simulink model "FlightSimulator_4160MODS"  (R2018a)
settings: Solver=FixedStepAuto  StartTime=0.0  StopTime=inf  RelTol=1e-3  EnableMultiTasking=on
undefined symbols (not defined in the file): LF, serial
libraries: aerolibutil x5, simulink x3, instrumentlib x3, sharedtransform x2, hdlsllib x1
settings Model: SimulationMode=accelerator  EnablePacing=on  PacingRate=1000  ExtModeTrigDuration=2  ExplicitPartitioning=on  Creator=argue  LastModifiedBy=User
settings OptimizationCC: EnhancedBackFolding=on  PassReuseOutputArgsAs=Individual arguments  MaxStackSize=64  OptimizeBlockOrder=speed  DifferentSizesBufferReuse=on  OptimizationCustomize=off
settings DebuggingCC: ParameterTunabilityLossMsg=error
settings HardwareCC: ProdBitPerPointer=32  ProdBitPerSizeT=32  ProdBitPerPtrDiffT=32  ProdLargestAtomicInteger=Long  ProdLargestAtomicFloat=Double  ProdWordSize=32  ProdHWDeviceType=ARM Compatible->ARM Cortex
settings SFSimCC: MATLABDynamicMemAlloc=off
settings RTWCC: SystemTargetFile=ert.tlc  HardwareBoard=Arduino Due  TLCOptions=-aInlineSetEventsForThisBaseRateFcn=TLC_FALSE -aSuppressMultiTaskScheduler=TLC_FALSE -aRateBasedStepFcn=1  TemplateMakefile=ert_default_tmf  GenerateReport=on  Toolchain=Arduino ARM  BuildConfiguration=Faster Runs  IncludeHyperlinkInReport=on  LaunchReport=on  GenerateTraceInfo=on  GenerateTraceReport=on  GenerateTraceReportSl=on  GenerateTraceReportSf=on  GenerateTraceReportEml=on
settings CodeAppCC: ForceParamTrailComments=on  IgnoreCustomStorageClasses=off  OperatorAnnotations=on  SimulinkDataObjDesc=on  SFDataObjDesc=on  InsertBlockDesc=on
settings ERTTargetCC: SupportContinuousTime=on  SupportVariableSizeSignals=on

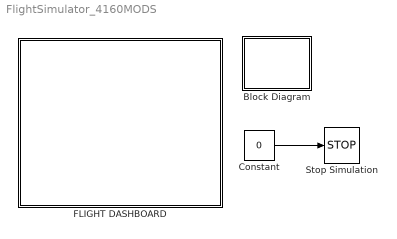
== system FlightSimulator_4160MODS ==
  Block Diagram : Subsystem
  Constant : Constant  Value=0
  FLIGHT DASHBOARD : Subsystem
  Stop Simulation : Stop
  wires:
  Constant/1 -> Stop Simulation/1

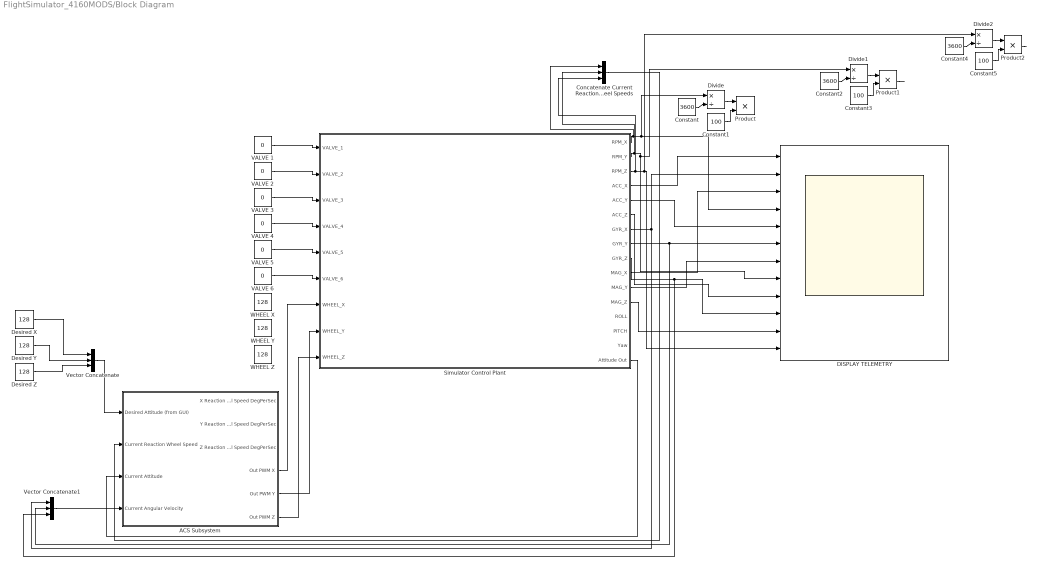
== system FlightSimulator_4160MODS/Block Diagram ==
  ACS Subsystem : Subsystem
  Concatenate Current Reaction Wheel Speeds : Concatenate  NumInputs=3
  Constant : Constant  Value=3600
  Constant1 : Constant  Value=100
  Constant2 : Constant  Value=3600
  Constant3 : Constant  Value=100
  Constant4 : Constant  Value=3600
  Constant5 : Constant  Value=100
  DISPLAY TELEMETRY : Scope  NumInputPorts=12
  Desired X : Constant  Value=128  OutDataTypeStr=double  SampleTime=-1
  Desired Y : Constant  Value=128  OutDataTypeStr=double  SampleTime=-1
  Desired Z : Constant  Value=128  OutDataTypeStr=double  SampleTime=-1
  Divide : Product  Inputs=*/
  Divide1 : Product  Inputs=*/
  Divide2 : Product  Inputs=*/
  Product : Product
  Product1 : Product
  Product2 : Product
  Simulator Control Plant : Subsystem
  VALVE {1..6} (6 alike) : Constant  Value=0  SampleTime=0.01
  Vector Concatenate : Concatenate  NumInputs=3
  Vector Concatenate1 : Concatenate  NumInputs=3
  WHEEL X : Constant  Value=128  OutDataTypeStr=int16  SampleTime=-1
  WHEEL Y : Constant  Value=128  OutDataTypeStr=int16  SampleTime=-1
  WHEEL Z : Constant  Value=128  OutDataTypeStr=int16  SampleTime=-1
  wires:
  VALVE 6/1 -> Simulator Control Plant/6(VALVE_6)
  VALVE 2/1 -> Simulator Control Plant/2(VALVE_2)
  VALVE 3/1 -> Simulator Control Plant/3(VALVE_3)
  VALVE 5/1 -> Simulator Control Plant/5(VALVE_5)
  VALVE 1/1 -> Simulator Control Plant/1(VALVE_1)
  VALVE 4/1 -> Simulator Control Plant/4(VALVE_4)
  Simulator Control Plant/4(" ACC_X") -> DISPLAY TELEMETRY/1
  Simulator Control Plant/7(GYR_X) -> Vector Concatenate1/1, DISPLAY TELEMETRY/2
  Simulator Control Plant/10(MAG_X) -> DISPLAY TELEMETRY/3
  Simulator Control Plant/1(RPM_X) -> Concatenate Current Reaction Wheel Speeds/1, Divide/1, DISPLAY TELEMETRY/4
  Simulator Control Plant/5(" ACC_Y") -> DISPLAY TELEMETRY/5
  Simulator Control Plant/8(GYR_Y) -> Vector Concatenate1/2, DISPLAY TELEMETRY/6
  Simulator Control Plant/11(MAG_Y) -> DISPLAY TELEMETRY/7
  Simulator Control Plant/6(" ACC_Z") -> DISPLAY TELEMETRY/9
  Simulator Control Plant/9(GYR_Z) -> Vector Concatenate1/3, DISPLAY TELEMETRY/10
  Simulator Control Plant/12(MAG_Z) -> DISPLAY TELEMETRY/11
  Constant/1 -> Divide/2
  Divide/1 -> Product/1
  Constant1/1 -> Product/2
  Simulator Control Plant/2(RPM_Y) -> Concatenate Current Reaction Wheel Speeds/2, Divide1/1, DISPLAY TELEMETRY/8
  Constant2/1 -> Divide1/2
  Divide1/1 -> Product1/1
  Constant3/1 -> Product1/2
  Divide2/1 -> Product2/1
  Constant4/1 -> Divide2/2
  Simulator Control Plant/3(RPM_Z) -> Concatenate Current Reaction Wheel Speeds/3, Divide2/1, DISPLAY TELEMETRY/12
  Constant5/1 -> Product2/2
  Product2/1 -> ?
  Product1/1 -> ?
  ACS Subsystem/6(Out PWM Z) -> Simulator Control Plant/9(WHEEL_Z)
  ACS Subsystem/5(Out PWM Y) -> Simulator Control Plant/8(WHEEL_Y)
  ACS Subsystem/4(Out PWM X) -> Simulator Control Plant/7(WHEEL_X)
  Concatenate Current Reaction Wheel Speeds/1 -> ACS Subsystem/2(Current Reaction Wheel Speed)
  Simulator Control Plant/16(" Attitude Out") -> ACS Subsystem/3(Current Attitude)
  Desired X/1 -> Vector Concatenate/1
  Desired Y/1 -> Vector Concatenate/2
  Desired Z/1 -> Vector Concatenate/3
  Vector Concatenate/1 -> ACS Subsystem/1(Desired Attitude (from GUI))
  Vector Concatenate1/1 -> ACS Subsystem/4(Current Angular Velocity)

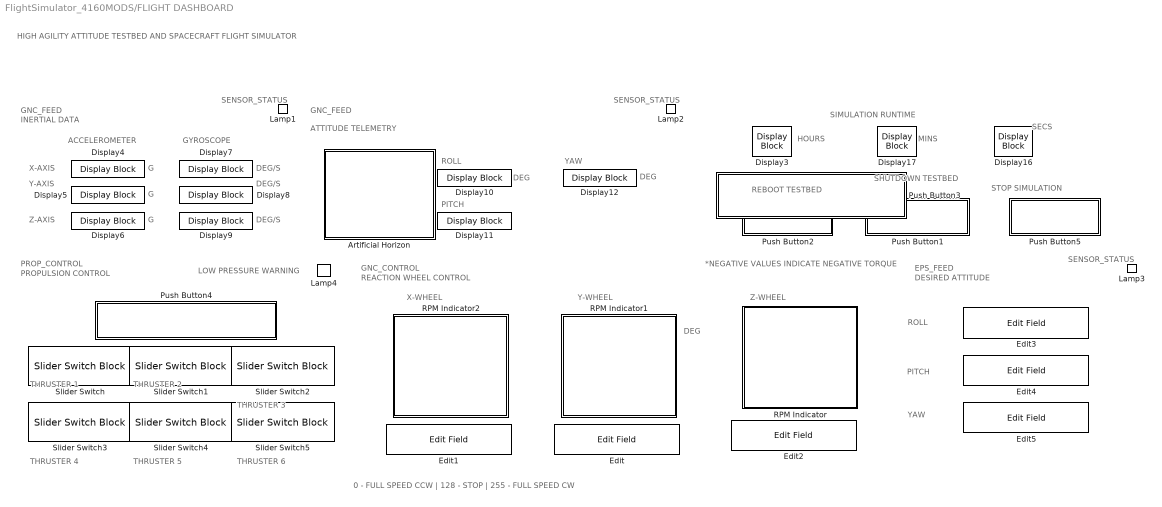
== system FlightSimulator_4160MODS/FLIGHT DASHBOARD ==
  note: HIGH AGILITY ATTITUDE TESTBED AND SPACECRAFT FLIGHT SIMULATOR
  note: PROPULSION CONTROL
  note: X-WHEEL
  note: LOW PRESSURE WARNING
  note: DESIRED ATTITUDE
  note: REACTION WHEEL CONTROL
  note: EPS_FEED
  note: PROP_CONTROL
  note: GNC_CONTROL
  note: GNC_FEED
  note: INERTIAL DATA
  note: G
  note: G
  note: G
  note: ACCELEROMETER
  note: X-AXIS
  note: Y-AXIS
  note: Z-AXIS
  note: GYROSCOPE
  note: DEG/S
  note: DEG/S
  note: DEG/S
  note: GNC_FEED
  note: ATTITUDE TELEMETRY
  note: ROLL
  note: PITCH
  note: YAW
  note: DEG
  note: DEG
  note: DEG
  note: SENSOR_STATUS
  note: SENSOR_STATUS
  note: SENSOR_STATUS
  note: *NEGATIVE VALUES INDICATE NEGATIVE TORQUE
  note: REBOOT TESTBED
  note: HOURS
  note: SECS
  note: MINS
  note: SIMULATION RUNTIME
  note: SHUTDOWN TESTBED
  note: STOP SIMULATION
  note: Y-WHEEL
  note: Z-WHEEL
  note: 0 - FULL SPEED CCW | 128 - STOP | 255 - FULL SPEED CW
  note: THRUSTER 1
  note: THRUSTER 2
  note: THRUSTER 3
  note: THRUSTER 4
  note: THRUSTER 6
  note: THRUSTER 5
  note: ROLL
  note: PITCH
  note: YAW
  Artificial Horizon : Subsystem  DialogController=aeroblksHMICreateDDGDialog  IsWebBlock=on  mask(MWDashboardBlock){webBlockId=87d256c6-158d-4fe2-b150-9c42d0428838, webBlockType=artificialhorizon, ShowInLibBrowser=on, ShowInitialText=on, HMISrcModelName=FlightSimulator}
      mask prompts: webBlockId "WebBlock Id"; webBlockType "WebBlock Type"; HMISrcModelName "Source Model"
      mask help: aeroblksHMI:aeroblkhmi:ArtificialHorizonDialogDesc
      mask Help: eval('asbhmihelp(''artificialhorizon'')');
      mask Display:
      | if strcmp(get_param(bdroot(gcb),'BlockDiagramType'), 'library')
      |  image([(matlabroot) '/toolbox/aeroblks/aeroblks/hmi/icons/ArtificialHorizonIcon.svg'])
      | end
  Display10 : DisplayBlock  WebBlockId=325  LabelPosition=Hide  Alignment=Left
  Display11 : DisplayBlock  WebBlockId=327  LabelPosition=Hide  Alignment=Left
  Display12 : DisplayBlock  WebBlockId=329  LabelPosition=Hide  Alignment=Left
  Display16 : DisplayBlock  WebBlockId=711  LabelPosition=Hide  Alignment=Left
  Display17 : DisplayBlock  WebBlockId=712  LabelPosition=Hide  Alignment=Left
  Display3 : DisplayBlock  WebBlockId=710  LabelPosition=Hide  Alignment=Left
  Display4 : DisplayBlock  WebBlockId=266  LabelPosition=Hide  Alignment=Left
  Display5 : DisplayBlock  WebBlockId=268  LabelPosition=Hide  Alignment=Left
  Display6 : DisplayBlock  WebBlockId=270  LabelPosition=Hide  Alignment=Left
  Display7 : DisplayBlock  WebBlockId=313  LabelPosition=Hide  Alignment=Left
  Display8 : DisplayBlock  WebBlockId=314  LabelPosition=Hide  Alignment=Left
  Display9 : DisplayBlock  WebBlockId=315  LabelPosition=Hide  Alignment=Left
  Edit : EditField  WebBlockId=830  LabelPosition=Hide  Alignment=Center
  Edit1 : EditField  WebBlockId=828  LabelPosition=Hide  Alignment=Center
  Edit2 : EditField  WebBlockId=829  LabelPosition=Hide  Alignment=Center
  Edit3 : EditField  WebBlockId=1336  LabelPosition=Hide  Alignment=Center
  Edit4 : EditField  WebBlockId=1337  LabelPosition=Hide  Alignment=Center
  Edit5 : EditField  WebBlockId=1338  LabelPosition=Hide  Alignment=Center
  Lamp1 : LampBlock  WebBlockId=841  LabelPosition=Hide
  Lamp2 : LampBlock  WebBlockId=399  LabelPosition=Hide
  Lamp3 : LampBlock  WebBlockId=401  LabelPosition=Hide
  Lamp4 : LampBlock  WebBlockId=1063  LabelPosition=Hide
  Push Button1 : Subsystem  DialogController=hmiCreateDDGDialog  IsWebBlock=on  mask(MWDashboardBlock){webBlockId=5529e01b-399f-4366-a248-23a197ffef9f, webBlockType=pushbutton, ShowInLibBrwoser=on, ShowInitialText=on, HMISrcModelName=FlightSimulator}
      mask prompts: webBlockId "WebBlock Id"; webBlockType "WebBlock Type"; HMISrcModelName "Source Model"
      mask help: SimulinkHMI:dialogs:PushButtonDialogDesc
      mask Help: helpview([docroot '/mapfiles/simulink.map'], 'hmi_push_button')
      mask Display:
      | model = bdroot(gcb);
      | if strcmp(get_param(model,'BlockDiagramType'), 'library')
      |     image([(matlabroot) '/toolbox/simulink/hmi/icons/PushButton.png']);
      | end
  Push Button2 : Subsystem  DialogController=hmiCreateDDGDialog  IsWebBlock=on  mask(MWDashboardBlock){webBlockId=2e9611f3-365a-4a15-a648-271fb47c7cf3, webBlockType=pushbutton, ShowInLibBrwoser=on, ShowInitialText=on, HMISrcModelName=FlightSimulator}
      mask prompts: webBlockId "WebBlock Id"; webBlockType "WebBlock Type"; HMISrcModelName "Source Model"
      mask help: SimulinkHMI:dialogs:PushButtonDialogDesc
      mask Help: helpview([docroot '/mapfiles/simulink.map'], 'hmi_push_button')
      mask Display:
      | model = bdroot(gcb);
      | if strcmp(get_param(model,'BlockDiagramType'), 'library')
      |     image([(matlabroot) '/toolbox/simulink/hmi/icons/PushButton.png']);
      | end
  Push Button3 : Subsystem  DialogController=hmiCreateDDGDialog  IsWebBlock=on  mask(MWDashboardBlock){webBlockId=2b20586d-f367-4741-bf9b-3cb173f58035, webBlockType=pushbutton, ShowInLibBrowser=on, ShowInitialText=on, HMISrcModelName=FlightSimulator}
      mask prompts: webBlockId "WebBlock Id"; webBlockType "WebBlock Type"; HMISrcModelName "Source Model"
      mask help: Set a value of a tunable parameter or variable by selecting and holding the button. When the push button is not selected, the value is set back to the default value.
      mask Help: helpview([docroot '/mapfiles/simulink.map'], 'hmi_pushbutton')
      mask Display:
      | if strcmp(get_param(bdroot(gcb),'BlockDiagramType'),'library')
      |  image([(matlabroot) '/toolbox/simulink/hmi/icons/PushButton.png'])
      | end
  Push Button4 : Subsystem  DialogController=hmiCreateDDGDialog  IsWebBlock=on  mask(MWDashboardBlock){webBlockId=373ea6f1-33bb-479d-964f-0db2d45018c2, webBlockType=pushbutton, ShowInLibBrwoser=on, ShowInitialText=on, HMISrcModelName=FlightSimulator}
      mask prompts: webBlockId "WebBlock Id"; webBlockType "WebBlock Type"; HMISrcModelName "Source Model"
      mask help: SimulinkHMI:dialogs:PushButtonDialogDesc
      mask Help: helpview([docroot '/mapfiles/simulink.map'], 'hmi_push_button')
      mask Display:
      | model = bdroot(gcb);
      | if strcmp(get_param(model,'BlockDiagramType'), 'library')
      |     image([(matlabroot) '/toolbox/simulink/hmi/icons/PushButton.png']);
      | end
  Push Button5 : Subsystem  DialogController=hmiCreateDDGDialog  IsWebBlock=on  mask(MWDashboardBlock){webBlockId=d7fbd1aa-2ff5-4984-a2a7-416a94e4d3e9, webBlockType=pushbutton, ShowInLibBrwoser=on, ShowInitialText=on, HMISrcModelName=FlightSimulator}
      mask prompts: webBlockId "WebBlock Id"; webBlockType "WebBlock Type"; HMISrcModelName "Source Model"
      mask help: SimulinkHMI:dialogs:PushButtonDialogDesc
      mask Help: helpview([docroot '/mapfiles/simulink.map'], 'hmi_push_button')
      mask Display:
      | model = bdroot(gcb);
      | if strcmp(get_param(model,'BlockDiagramType'), 'library')
      |     image([(matlabroot) '/toolbox/simulink/hmi/icons/PushButton.png']);
      | end
  RPM Indicator : Subsystem  DialogController=aeroblksHMICreateDDGDialog  IsWebBlock=on  mask(MWDashboardBlock){webBlockId=08a9e829-d632-43db-b174-ac85f5d525a0, webBlockType=rpmindicator, ShowInLibBrowser=on, ShowInitialText=on, HMISrcModelName=FlightSimulator}
      mask prompts: webBlockId "WebBlock Id"; webBlockType "WebBlock Type"; HMISrcModelName "Source Model"
      mask help: aeroblksHMI:aeroblkhmi:RPMIndicatorDialogDesc
      mask Help: eval('asbhmihelp(''rpmindicator'')')
      mask Display:
      | if strcmp(get_param(bdroot(gcb),'BlockDiagramType'), 'library')
      |  image([(matlabroot) '/toolbox/aeroblks/aeroblks/hmi/icons/RPMIndicatorIcon.svg'])
      | end
  RPM Indicator1 : Subsystem  DialogController=aeroblksHMICreateDDGDialog  IsWebBlock=on  mask(MWDashboardBlock){webBlockId=8ce8b2ac-7bb7-4973-85b6-cdafd251f30d, webBlockType=rpmindicator, ShowInLibBrowser=on, ShowInitialText=on, HMISrcModelName=FlightSimulator}
      mask prompts: webBlockId "WebBlock Id"; webBlockType "WebBlock Type"; HMISrcModelName "Source Model"
      mask help: aeroblksHMI:aeroblkhmi:RPMIndicatorDialogDesc
      mask Help: eval('asbhmihelp(''rpmindicator'')')
      mask Display:
      | if strcmp(get_param(bdroot(gcb),'BlockDiagramType'), 'library')
      |  image([(matlabroot) '/toolbox/aeroblks/aeroblks/hmi/icons/RPMIndicatorIcon.svg'])
      | end
  RPM Indicator2 : Subsystem  DialogController=aeroblksHMICreateDDGDialog  IsWebBlock=on  mask(MWDashboardBlock){webBlockId=a80f6973-3156-4565-aff3-9397dcdba22e, webBlockType=rpmindicator, ShowInLibBrowser=on, ShowInitialText=on, HMISrcModelName=FlightSimulator}
      mask prompts: webBlockId "WebBlock Id"; webBlockType "WebBlock Type"; HMISrcModelName "Source Model"
      mask help: aeroblksHMI:aeroblkhmi:RPMIndicatorDialogDesc
      mask Help: eval('asbhmihelp(''rpmindicator'')')
      mask Display:
      | if strcmp(get_param(bdroot(gcb),'BlockDiagramType'), 'library')
      |  image([(matlabroot) '/toolbox/aeroblks/aeroblks/hmi/icons/RPMIndicatorIcon.svg'])
      | end
  Slider Switch : SliderSwitchBlock  WebBlockId=1066
      settings: Values={{'Off', 'On'}, [0 1]}
  Slider Switch1 : SliderSwitchBlock  WebBlockId=1067
      settings: Values={{'Off', 'On'}, [0 1]}
  Slider Switch2 : SliderSwitchBlock  WebBlockId=1068
      settings: Values={{'Off', 'On'}, [0 1]}
  Slider Switch3 : SliderSwitchBlock  WebBlockId=1069
      settings: Values={{'Off', 'On'}, [0 1]}
  Slider Switch4 : SliderSwitchBlock  WebBlockId=1070
      settings: Values={{'Off', 'On'}, [0 1]}
  Slider Switch5 : SliderSwitchBlock  WebBlockId=1071
      settings: Values={{'Off', 'On'}, [0 1]}

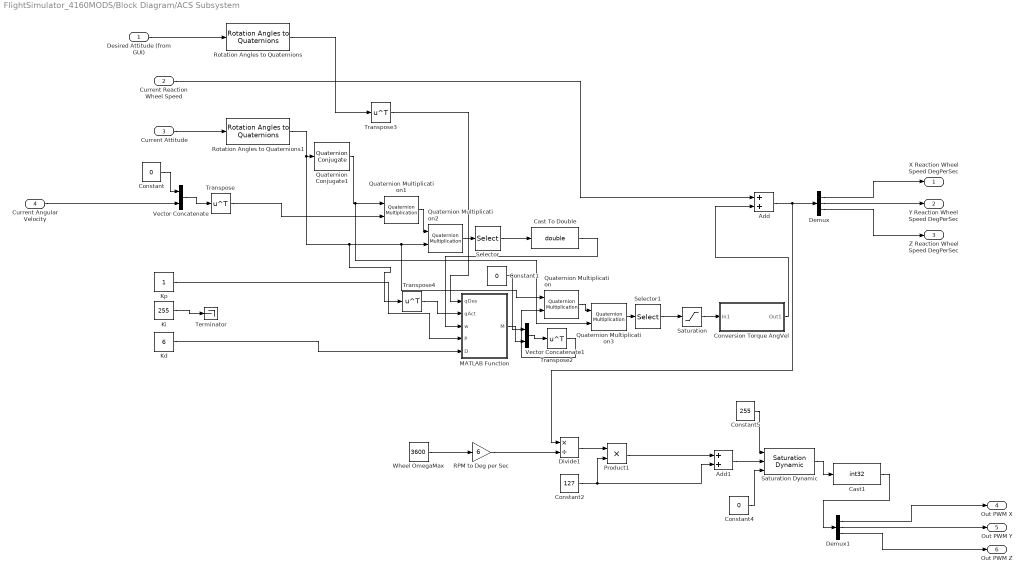
== system FlightSimulator_4160MODS/Block Diagram/ACS Subsystem ==
  Desired Attitude (from GUI) : Inport
  Current Reaction Wheel Speed : Inport  Port=2
  Current Attitude : Inport  Port=3
  Current Angular Velocity : Inport  Port=4
  Add : Sum
  Add1 : Sum
  Cast To Double : DataTypeConversion  OutDataTypeStr=double
  Cast1 : DataTypeConversion  OutDataTypeStr=int32  SaturateOnIntegerOverflow=on
  Constant : Constant  Value=0
  Constant1 : Constant  Value=0
  Constant2 : Constant  Value=127
  Constant4 : Constant  Value=0
  Constant5 : Constant  Value=255
  Conversion Torque AngVel : Subsystem
  Demux : Demux  Outputs=3
  Demux1 : Demux  Outputs=3
  Divide1 : Product  Inputs=*/
  Kd : Constant  Value=6  OutDataTypeStr=double  SampleTime=-1
  Ki : Constant  Value=255  OutDataTypeStr=double  SampleTime=-1
  Kp : Constant  OutDataTypeStr=double  SampleTime=-1
  MATLAB Function : MATLAB Function  TreatAsAtomicUnit=on
  Product1 : Product
  Quaternion Conjugate1 : aerolibutil/Quaternion Conjugate
      settings: SourceProductName=Aerospace Blockset  SourceProductBaseCode=AE
  Quaternion Multiplication{,1..3} (4 alike) : aerolibutil/Quaternion Multiplication
  RPM to Deg per Sec : Gain  Gain=6
  Rotation Angles to Quaternions : sharedtransform/Rotation Angles to Quaternions  rotationOrder=XYZ  aMode=aMode
      settings: SourceProductName=Aerospace Blockset  SourceProductBaseCode=AE
  Rotation Angles to Quaternions1 : sharedtransform/Rotation Angles to Quaternions  rotationOrder=XYZ  aMode=aMode
      settings: SourceProductName=Aerospace Blockset  SourceProductBaseCode=AE
  Saturation : Saturate  UpperLimit=0.43  LowerLimit=-0.43
  Saturation Dynamic : simulink/Discontinuities/Saturation Dynamic  OutMin=[]  OutMax=[]  OutDataTypeStr=Inherit: Same as second input  OutDataType=fixdt(1, 16)  OutScaling=2^-10  DoSatur=off
  Selector : Selector  InputPortWidth=4  IndexOptions=Index vector (dialog)  Indices=[2 3 4]  OutputSizes=1
  Selector1 : Selector  InputPortWidth=4  IndexOptions=Index vector (dialog)  Indices=[2 3 4]  OutputSizes=1
  Terminator : Terminator
  Transpose{,2..4} (4 alike) : Math  Operator=transpose  SaturateOnIntegerOverflow=on
  Vector Concatenate : Concatenate
  Vector Concatenate1 : Concatenate
  Wheel OmegaMax : Constant  Value=3600
  X Reaction Wheel Speed DegPerSec : Outport
  Y Reaction Wheel Speed DegPerSec : Outport  Port=2
  Z Reaction Wheel Speed DegPerSec : Outport  Port=3
  Out PWM X : Outport  Port=4
  Out PWM Y : Outport  Port=5
  Out PWM Z : Outport  Port=6
  wires:
  Constant4/1 -> Saturation Dynamic/3
  Kd/1 -> MATLAB Function/5(D)
  Kp/1 -> MATLAB Function/4(P)
  Demux/3 -> Z Reaction Wheel Speed DegPerSec/1
  Constant5/1 -> Saturation Dynamic/1
  Product1/1 -> Add1/1
  Divide1/1 -> Product1/1
  Demux/1 -> X Reaction Wheel Speed DegPerSec/1
  Wheel OmegaMax/1 -> RPM to Deg per Sec/1
  Demux/2 -> Y Reaction Wheel Speed DegPerSec/1
  Demux1/2 -> Out PWM Y/1
  Demux1/3 -> Out PWM Z/1
  Current Attitude/1 -> Rotation Angles to Quaternions1/1
  Demux1/1 -> Out PWM X/1
  Desired Attitude (from GUI)/1 -> Rotation Angles to Quaternions/1
  Conversion Torque AngVel/1(Out1) -> Add/2
  Add/1 -> Divide1/1, Demux/1
  Current Reaction Wheel Speed/1 -> Add/1
  Rotation Angles to Quaternions1/1 -> Transpose4/1, Quaternion Multiplication/1, Quaternion Multiplication2/2, Quaternion Conjugate1/1
  Current Angular Velocity/1 -> Vector Concatenate/2
  Constant/1 -> Vector Concatenate/1
  Vector Concatenate/1 -> Transpose/1
  Transpose/1 -> Quaternion Multiplication1/2
  Quaternion Multiplication1/1 -> Quaternion Multiplication2/1
  Quaternion Conjugate1/1 -> Quaternion Multiplication3/2, Quaternion Multiplication1/1
  Quaternion Multiplication2/1 -> Selector/1
  Selector/1 -> Cast To Double/1
  Ki/1 -> Terminator/1
  Constant1/1 -> Vector Concatenate1/1
  MATLAB Function/1(M) -> Vector Concatenate1/2
  Vector Concatenate1/1 -> Transpose2/1
  Transpose2/1 -> Quaternion Multiplication/2
  Quaternion Multiplication/1 -> Quaternion Multiplication3/1
  Quaternion Multiplication3/1 -> Selector1/1
  Selector1/1 -> Saturation/1
  RPM to Deg per Sec/1 -> Divide1/2
  Rotation Angles to Quaternions/1 -> Transpose3/1
  Transpose3/1 -> MATLAB Function/1(qDes)
  Transpose4/1 -> MATLAB Function/2(qAct)
  Constant2/1 -> Add1/2, Product1/2
  Add1/1 -> Saturation Dynamic/2
  Saturation Dynamic/1 -> Cast1/1
  Cast1/1 -> Demux1/1
  Cast To Double/1 -> MATLAB Function/3(w)
  Saturation/1 -> Conversion Torque AngVel/1(In1)

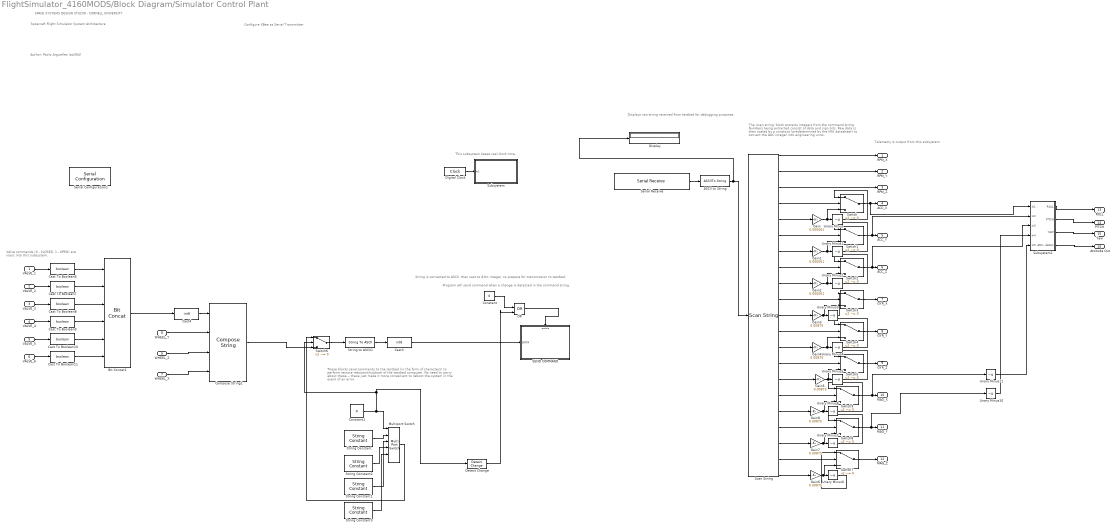
== system FlightSimulator_4160MODS/Block Diagram/Simulator Control Plant ==
  note: Spcecraft Flight Simulator System Architecture
  note: Configure XBee as Serial Transmitter
  note: Valve commands (0 - CLOSED, 1 - OPEN) are input into this subsystem.
  note: The 'scan string' block extracts integers from the command string. Numbers being extracted consist of data and sign bits. Raw data is then scaled by a constant (predetermined by the IMU datasheet) to convert the ADC integer into engineering units.
  note: This subsystem keeps real clock time.
  note: These blocks send commands to the testbed (in the form of characters) to perform remote reboots/shutdown of the testbed computer. No need to worry about these -- these just make it more convenient to reboot the system in the event of an error.
  note: String is converted to ASCII, then cast to 8-bit integer, to prepare for transmission to testbed.
  note: Program will send command when a change is detected in the command string.
  note: Displays raw string received from testbed for debugging purposes.
  note: Telemetry is output from this subsystem.
  note: Author: Paolo Arguelles (pa394)
  note: SPACE SYSTEMS DESIGN STUDIO - CORNELL UNIVERSITY
  VALVE_1 : Inport
  VALVE_2 : Inport  Port=2
  VALVE_3 : Inport  Port=3
  VALVE_4 : Inport  Port=4
  VALVE_5 : Inport  Port=5
  VALVE_6 : Inport  Port=6
  WHEEL_X : Inport  Port=7
  WHEEL_Y : Inport  Port=8
  WHEEL_Z : Inport  Port=9
  ASCII to String : ASCIIToString
  Bit Concat1 : hdlsllib/Logic and Bit Operations/Bit Concat  numInputs=6
      settings: SourceProductName=HDL Coder  SourceProductBaseCode=HD
  Cast To Boolean{6..11} (6 alike) : DataTypeConversion  OutDataTypeStr=boolean
  Cast3 : DataTypeConversion  OutDataTypeStr=int8
  Cast4 : DataTypeConversion  OutDataTypeStr=int8
  Compose String1 : ComposeString  Format="\"%d;%d;%d;%d\\n\""
  Constant : Constant  Value=0
  Constant1 : Constant  Value=0  VectorParams1D=off  SampleTime=-1
  Detect Change : simulink/Logic and Bit Operations/Detect Change  vinit=0  OutDataTypeStr=boolean
  Digital Clock : DigitalClock  SampleTime=-1
  Display : Display
  Gain : Gain  Gain=0.000061  OutDataTypeStr=double
  Gain1 : Gain  Gain=0.000061  OutDataTypeStr=double
  Gain2 : Gain  Gain=0.000061  OutDataTypeStr=double
  Gain{3..5,7..8} (5 alike) : Gain  Gain=0.00875  OutDataTypeStr=double
  Gain6 : Gain  Gain=0.00875
  Multiport Switch : MultiPortSwitch  Inputs=5  DiagnosticForDefault=None
  OR : Logic  Operator=OR  IconShape=distinctive  AllPortsSameDT=off  OutDataTypeStr=boolean
  SEND COMMAND : Subsystem
  Scan String : ScanString  Format="\"\\n%d;%d;%d$%d$%d$%d$%d$%d$%d$%d$%d$%d$%d$%d$%d$%d$%d$%d$%d$%d$%d\\r\""
  Serial Configuration1 : instrumentlib/Serial Configuration  Priority=-200000  ComPortMenu=COM5  ComPort=COM5  ObjConstructor=serial('COM5');  BaudRate=9600  DataBits=8  Parity=none  StopBits=1  FlowControl=none  Timeout=5  ByteOrder=LittleEndian
  Serial Receive : instrumentlib/Serial Receive  ComPortMenu=COM5  ComPort=COM5  ObjConstructor=serial('COM5');  Header=\r  Terminator=LF ('\n')  DataSize=88  DataType=uint8  EnableBlockingMode=on  ActionDataUnavailable=Output custom value  CustomValue=0  SampleTime=-1
  String Constant : StringConstant  String='Q'
  String Constant1 : StringConstant  String='R'
  String Constant2 : StringConstant  String='S'
  String Constant3 : StringConstant  String='B'
  String to ASCII1 : StringToASCII  MaximumLength=27
  Subsystem : Subsystem
  Subsystem1 : Subsystem
  Switch{,1..9} (10 alike) : Switch  Criteria=u2 ~= 0
  Unary Minus{,1..8,10..11} (11 alike) : UnaryMinus
  RPM_X : Outport
  RPM_Y : Outport  Port=2
  RPM_Z : Outport  Port=3
  " ACC_X" : Outport  Port=4
  " ACC_Y" : Outport  Port=5
  " ACC_Z" : Outport  Port=6
  GYR_X : Outport  Port=7
  GYR_Y : Outport  Port=8
  GYR_Z : Outport  Port=9
  MAG_X : Outport  Port=10
  MAG_Y : Outport  Port=11
  MAG_Z : Outport  Port=12
  " ROLL" : Outport  Port=13
  " PITCH" : Outport  Port=14
  " Yaw" : Outport  Port=15
  " Attitude Out" : Outport  Port=16
  wires:
  Gain1/1 -> Switch1/3, Unary Minus1/1
  Scan String/7 -> Gain1/1
  Unary Minus/1 -> Switch/1
  ASCII to String/1 -> Display/1, Scan String/1
  Unary Minus5/1 -> Switch5/1
  Gain4/1 -> Switch4/3, Unary Minus4/1
  Scan String/6 -> Switch1/2
  Scan String/11 -> Gain3/1
  Cast To Boolean6/1 -> Bit Concat1/1
  String Constant2/1 -> Multiport Switch/4
  Switch5/1 -> GYR_Z/1
  Gain/1 -> Switch/3, Unary Minus/1
  Switch3/1 -> GYR_X/1
  Gain3/1 -> Switch3/3, Unary Minus3/1
  Scan String/1 -> RPM_X/1
  Switch4/1 -> GYR_Y/1
  Scan String/8 -> Switch2/2
  Compose String1/1 -> Switch6/3
  Cast To Boolean11/1 -> Bit Concat1/6
  VALVE_4/1 -> Cast To Boolean9/1
  Bit Concat1/1 -> Cast4/1
  Switch6/1 -> String to ASCII1/1
  Cast To Boolean8/1 -> Bit Concat1/3
  Scan String/13 -> Gain4/1
  Scan String/14 -> Switch5/2
  Cast To Boolean10/1 -> Bit Concat1/5
  Scan String/4 -> Switch/2
  Cast To Boolean9/1 -> Bit Concat1/4
  Scan String/12 -> Switch4/2
  Switch/1 -> Subsystem1/1(In1), " ACC_X"/1
  Cast To Boolean7/1 -> Bit Concat1/2
  Gain5/1 -> Switch5/3, Unary Minus5/1
  Scan String/10 -> Switch3/2
  Scan String/9 -> Gain2/1
  Unary Minus2/1 -> Switch2/1
  VALVE_5/1 -> Cast To Boolean10/1
  Gain2/1 -> Switch2/3, Unary Minus2/1
  Unary Minus4/1 -> Switch4/1
  Unary Minus1/1 -> Switch1/1
  VALVE_1/1 -> Cast To Boolean6/1
  Scan String/2 -> RPM_Y/1
  Scan String/3 -> RPM_Z/1
  Switch1/1 -> Subsystem1/2(In2), " ACC_Y"/1
  Switch2/1 -> Subsystem1/3(In3), " ACC_Z"/1
  Unary Minus3/1 -> Switch3/1
  Scan String/5 -> Gain/1
  VALVE_2/1 -> Cast To Boolean7/1
  Digital Clock/1 -> Subsystem/1(In1)
  Serial Receive/1 -> ASCII to String/1
  String Constant/1 -> Multiport Switch/2
  VALVE_3/1 -> Cast To Boolean8/1
  String to ASCII1/1 -> Cast3/1
  VALVE_6/1 -> Cast To Boolean11/1
  String Constant3/1 -> Multiport Switch/5
  Multiport Switch/1 -> Switch6/1
  String Constant1/1 -> Multiport Switch/3
  Scan String/15 -> Gain5/1
  Gain6/1 -> Switch7/3, Unary Minus6/1
  Scan String/21 -> Gain6/1
  Scan String/20 -> Switch7/2
  Unary Minus6/1 -> Switch7/1
  Unary Minus7/1 -> Switch8/1
  Scan String/19 -> Gain7/1
  Scan String/18 -> Switch8/2
  Gain7/1 -> Switch8/3, Unary Minus7/1
  Unary Minus8/1 -> Switch9/1
  Scan String/17 -> Gain8/1
  Scan String/16 -> Switch9/2
  Gain8/1 -> Switch9/3, Unary Minus8/1
  Switch7/1 -> MAG_Z/1
  Switch8/1 -> Unary Minus10/1, MAG_Y/1
  Switch9/1 -> Unary Minus11/1, MAG_X/1
  Cast4/1 -> Compose String1/1
  Subsystem1/1(" ROLL") -> " ROLL"/1
  Subsystem1/2(" PITCH") -> " PITCH"/1
  WHEEL_Y/1 -> Compose String1/2
  WHEEL_Z/1 -> Compose String1/3
  WHEEL_X/1 -> Compose String1/4
  Detect Change/1 -> OR/2
  Constant1/1 -> Detect Change/1, Switch6/2, Multiport Switch/1
  Constant/1 -> OR/1
  OR/1 -> SEND COMMAND/Enable
  Cast3/1 -> SEND COMMAND/1(DATA)
  Unary Minus10/1 -> Subsystem1/4(In4)
  Unary Minus11/1 -> Subsystem1/5(In5)
  Subsystem1/3(" YAW") -> " Yaw"/1
  Subsystem1/4(" AttitudeOut") -> " Attitude Out"/1

== system FlightSimulator_4160MODS/FLIGHT DASHBOARD/Artificial Horizon ==

== system FlightSimulator_4160MODS/FLIGHT DASHBOARD/Push Button1 ==

== system FlightSimulator_4160MODS/FLIGHT DASHBOARD/Push Button2 ==

== system FlightSimulator_4160MODS/FLIGHT DASHBOARD/Push Button3 ==

== system FlightSimulator_4160MODS/FLIGHT DASHBOARD/Push Button4 ==

== system FlightSimulator_4160MODS/FLIGHT DASHBOARD/Push Button5 ==

== system FlightSimulator_4160MODS/FLIGHT DASHBOARD/RPM Indicator ==

== system FlightSimulator_4160MODS/FLIGHT DASHBOARD/RPM Indicator1 ==

== system FlightSimulator_4160MODS/FLIGHT DASHBOARD/RPM Indicator2 ==

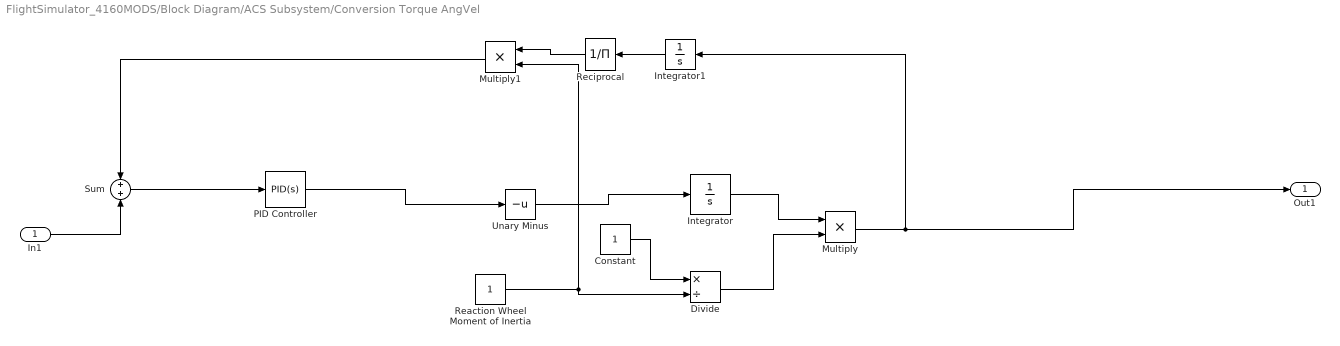
== system FlightSimulator_4160MODS/Block Diagram/ACS Subsystem/Conversion Torque AngVel ==
  In1 : Inport
  Constant : Constant
  Divide : Product  Inputs=*/
  Integrator : Integrator
  Integrator1 : Integrator
  Multiply : Product
  Multiply1 : Product
  PID Controller : simulink/Continuous/PID Controller  Controller=PID  TimeDomain=Continuous-time  SampleTime=-1  IntegratorMethod=Forward Euler  FilterMethod=Forward Euler  Form=Parallel  UseFilter=on  ControllerParametersSource=internal  P=10  I=0.01  D=20  N=100  InitialConditionSource=internal  InitialConditionForIntegrator=0  InitialConditionForFilter=0  ExternalReset=none  LimitOutput=off  UpperSaturationLimit=inf  LowerSaturationLimit=-inf  LinearizeAsGain=on  AntiWindupMode=none  Kb=1  TrackingMode=off  Kt=1  PParamMin=[]  PParamMax=[]  IParamMin=[]  IParamMax=[]  DParamMin=[]  DParamMax=[]  NParamMin=[]  NParamMax=[]  KbParamMin=[]  KbParamMax=[]  KtParamMin=[]  KtParamMax=[]  POutMin=[]  POutMax=[]  IOutMin=[]  IOutMax=[]  DOutMin=[]  DOutMax=[]  NOutMin=[]  NOutMax=[]  KbOutMin=[]  KbOutMax=[]  KtOutMin=[]  KtOutMax=[]  IntegratorOutMin=[]  IntegratorOutMax=[]  FilterOutMin=[]  FilterOutMax=[]  SumOutMin=[]  SumOutMax=[]  SumI1OutMin=[]  SumI1OutMax=[]  SumI2OutMin=[]  SumI2OutMax=[]  SumI3OutMin=[]  SumI3OutMax=[]  SumDOutMin=[]  SumDOutMax=[]  SaturationOutMin=[]  SaturationOutMax=[]  IntegratorContinuousStateAttributes=''  IntegratorStateMustResolveToSignalObject=off  IntegratorRTWStateStorageClass=Auto  FilterContinuousStateAttributes=''  FilterStateMustResolveToSignalObject=off  FilterRTWStateStorageClass=Auto  DifferentiatorICPrevScaledInput=0  DifferentiatorOutMin=[]  DifferentiatorOutMax=[]  FilterDiffOutCoefMin=[]  FilterDiffOutCoefMax=[]  SumDenOutMin=[]  SumDenOutMax=[]  SumNumOutMin=[]  SumNumOutMax=[]  ReciprocalOutMin=[]  ReciprocalOutMax=[]  DivideOutMin=[]  DivideOutMax=[]  TunerSelectOption=Transfer Function Based (PID Tuner App)
  Reaction Wheel Moment of Inertia : Constant
  Reciprocal : Product  Inputs=/
  Sum : Sum  Inputs=+|+
  Unary Minus : UnaryMinus
  Out1 : Outport
  wires:
  PID Controller/1 -> Unary Minus/1
  Unary Minus/1 -> Integrator/1
  Constant/1 -> Divide/1
  Reaction Wheel Moment of Inertia/1 -> Multiply1/2, Divide/2
  Integrator/1 -> Multiply/1
  Divide/1 -> Multiply/2
  Multiply/1 -> Integrator1/1, Out1/1
  Integrator1/1 -> Reciprocal/1
  Reciprocal/1 -> Multiply1/1
  In1/1 -> Sum/2
  Multiply1/1 -> Sum/1
  Sum/1 -> PID Controller/1

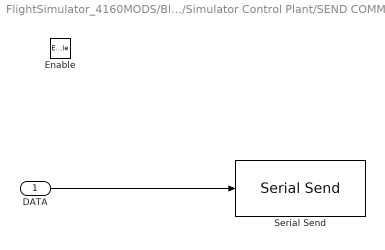
== system FlightSimulator_4160MODS/Block Diagram/Simulator Control Plant/SEND COMMAND ==
  DATA : Inport
  Enable : EnablePort  ShowOutputPort=on
  Serial Send : instrumentlib/Serial Send  ComPortMenu=COM5  ComPort=COM5  ObjConstructor=serial('COM5');  Terminator=<none>  EnableBlockingMode=on
  wires:
  DATA/1 -> Serial Send/1

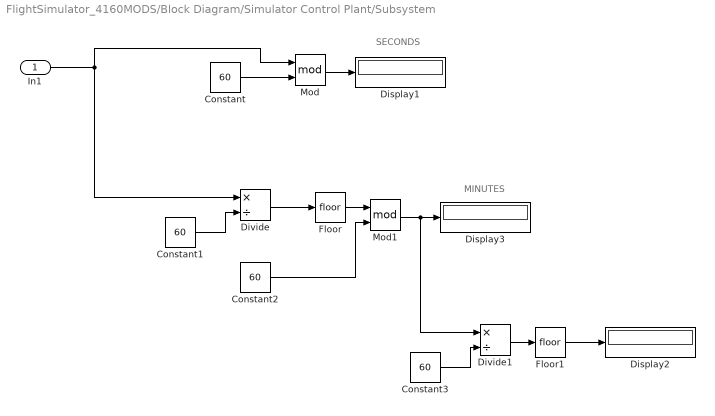
== system FlightSimulator_4160MODS/Block Diagram/Simulator Control Plant/Subsystem ==
  note: SECONDS
  note: MINUTES
  In1 : Inport
  Constant{,1..3} (4 alike) : Constant  Value=60
  Display1 : Display
  Display2 : Display
  Display3 : Display
  Divide : Product  Inputs=*/
  Divide1 : Product  Inputs=*/
  Floor : Rounding
  Floor1 : Rounding
  Mod : Math  Operator=mod  SaturateOnIntegerOverflow=on
  Mod1 : Math  Operator=mod  SaturateOnIntegerOverflow=on
  wires:
  Constant/1 -> Mod/2
  Mod/1 -> Display1/1
  In1/1 -> Divide/1, Mod/1
  Constant1/1 -> Divide/2
  Divide/1 -> Floor/1
  Floor/1 -> Mod1/1
  Constant2/1 -> Mod1/2
  Mod1/1 -> Divide1/1, Display3/1
  Constant3/1 -> Divide1/2
  Divide1/1 -> Floor1/1
  Floor1/1 -> Display2/1

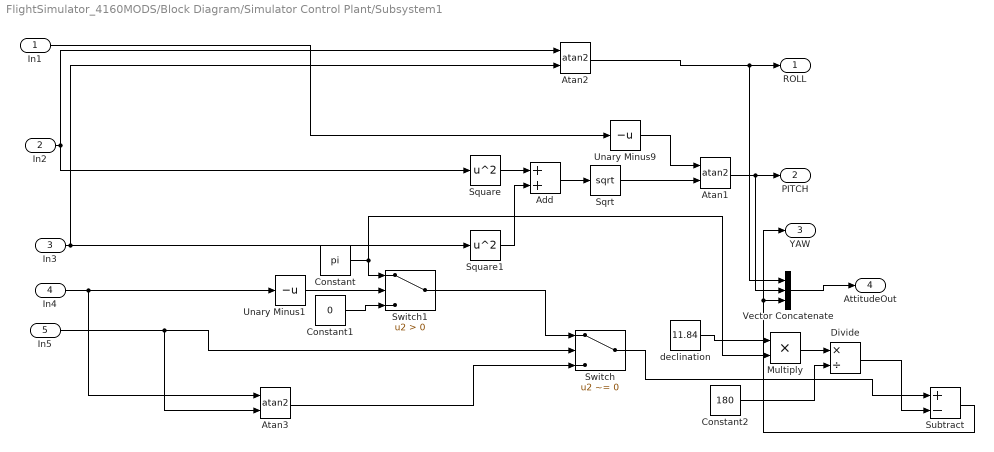
== system FlightSimulator_4160MODS/Block Diagram/Simulator Control Plant/Subsystem1 ==
  In1 : Inport
  In2 : Inport  Port=2
  In3 : Inport  Port=3
  In4 : Inport  Port=4
  In5 : Inport  Port=5
  Add : Sum
  Atan1 : Trigonometry  Operator=atan2
  Atan2 : Trigonometry  Operator=atan2  OutputSignalType=real
  Atan3 : Trigonometry  Operator=atan2
  Constant : Constant  Value=pi
  Constant1 : Constant  Value=0
  Constant2 : Constant  Value=180
  Divide : Product  Inputs=*/
  Multiply : Product
  Sqrt : Sqrt  SaturateOnIntegerOverflow=on
  Square : Math  Operator=square  SaturateOnIntegerOverflow=on
  Square1 : Math  Operator=square  SaturateOnIntegerOverflow=on
  Subtract : Sum  Inputs=+-
  Switch : Switch  Criteria=u2 ~= 0
  Switch1 : Switch  Criteria=u2 > Threshold
  Unary Minus1 : UnaryMinus
  Unary Minus9 : UnaryMinus
  Vector Concatenate : Concatenate  NumInputs=3
  declination : Constant  Value=11.84
  " ROLL" : Outport
  " PITCH" : Outport  Port=2
  " YAW" : Outport  Port=3
  " AttitudeOut" : Outport  Port=4
  wires:
  Square1/1 -> Add/2
  Sqrt/1 -> Atan1/2
  Unary Minus9/1 -> Atan1/1
  Atan1/1 -> Vector Concatenate/2, " PITCH"/1
  Atan2/1 -> Vector Concatenate/1, " ROLL"/1
  In2/1 -> Square/1, Atan2/1
  Square/1 -> Add/1
  Add/1 -> Sqrt/1
  In1/1 -> Unary Minus9/1
  In3/1 -> Square1/1, Atan2/2
  In5/1 -> Atan3/2, Switch/2
  In4/1 -> Atan3/1, Unary Minus1/1
  Unary Minus1/1 -> Switch1/2
  Constant/1 -> Multiply/2, Switch1/1
  Constant1/1 -> Switch1/3
  Switch1/1 -> Switch/1
  Atan3/1 -> Switch/3
  declination/1 -> Multiply/1
  Multiply/1 -> Divide/1
  Constant2/1 -> Divide/2
  Switch/1 -> Subtract/1
  Divide/1 -> Subtract/2
  Subtract/1 -> " YAW"/1, Vector Concatenate/3
  Vector Concatenate/1 -> " AttitudeOut"/1

== matlab function FlightSimulator_4160MODS/Block Diagram/ACS Subsystem/MATLAB Function ==
  data: qDes input; M output; qAct input; w input; P input; D input
function M=controlAlg2(qDes,qAct,w,P,D)
    qErr=quatmultiply(quatconj(qDes), qAct);
    
    sinTheta=norm(qErr(2:4)); cosTheta=qErr(1);
    theta=2*atan2(sinTheta,cosTheta);
    if ~sinTheta==0
        axisVect=qErr(2:4)'/sinTheta;
    else
        axisVect=[0;0;0];
    end
    if theta>pi
        theta=theta-2*pi;
    end
    
    dw=-P*axisVect*theta-D*w;
    M=6*dw;
    
end
